simulink model "IBR_Control_Benchmark_2024b"  (R2024b)
settings: Solver=ode4  StartTime=0.0  StopTime=1  FixedStep=5e-5  RelTol=1e-3
values from neighbouring files (symbols this model uses):
  Ki_I = Simulink.Parameter    [IBR_Control_Parameters.m]
  Ki_PLL = Simulink.Parameter    [IBR_Control_Parameters.m]
  Kp_I = Simulink.Parameter    [IBR_Control_Parameters.m]
  Kp_PLL = Simulink.Parameter    [IBR_Control_Parameters.m]
  Lc = Simulink.Parameter    [IBR_Control_Parameters.m]
  Pref = Simulink.Parameter    [IBR_Control_Parameters.m]
  Qref = Simulink.Parameter    [IBR_Control_Parameters.m]
  Rc = Simulink.Parameter    [IBR_Control_Parameters.m]
  Re = Vn^2 / Sk / sqrt(RXratio^2 + 1) * RXratio    [IBR_Control_Parameters.m]
  Vn = 400e3    (= 400000)    [IBR_Control_Parameters.m]
undefined symbols (not defined in the file or in its folder): cVc, DiscIntNeverNeededParam, dspblkCoreblockFVToolHelper, fn, gcbh, ia0, ib0, ic0, id0, iq0, Kp_S, Le, T_S, theta0
libraries: slpidlib x3, model_info x1
settings Model: ParamWorkspaceSource=ReferencedWorkspace  Creator=evansolingen  LastModifiedBy=if47izeq
settings DataIOCC: LimitDataPoints=on  SaveFormat=Array  SignalLoggingSaveFormat=ModelDataLogs  SaveOutput=off  SignalLogging=off  SaveTime=off  ReturnWorkspaceOutputs=off
settings OptimizationCC: EnhancedBackFolding=on  ExpressionFolding=off  PassReuseOutputArgsThreshold=0  ExpressionDepthLimit=2147483647  OptimizeBlockOrder=speed  DifferentSizesBufferReuse=on
settings DebuggingCC: UnderspecifiedInitializationDetection=Classic  MergeDetectMultiDrivingBlocksExec=none  SolverPrmCheckMsg=warning  MultiTaskDSMMsg=warning  MultiTaskCondExecSysMsg=none  ParameterTunabilityLossMsg=error  FcnCallInpInsideContextMsg=warning  UnconnectedInputMsg=warning  UnconnectedOutputMsg=warning  UnconnectedLineMsg=warning  AllowSymbolicDim=off  StateNameClashWarn=warning  SFUnexpectedBacktrackingDiag=warning  SFNoUnconditionalDefaultTransitionDiag=warning  SFExecutionAtInitializationDiag=none  UnderSpecifiedDimensionMsg=warning  ArithmeticOperatorsInVariantConditions=warning
settings HardwareCC: ProdBitPerPointer=32  ProdBitPerSizeT=32  ProdBitPerPtrDiffT=32  ProdLargestAtomicFloat=None  ProdIntDivRoundTo=Undefined  ProdEndianess=Unspecified  ProdWordSize=32  ProdHWDeviceType=32-bit Generic
settings ModelReferenceCC: UpdateModelReferenceTargets=Force  EnableRefExpFcnMdlSchedulingChecks=on  PropagateSignalLabelsOutOfModel=off
settings SFSimCC: SimUseLocalCustomCode=off  SimParseCustomCode=off  MATLABDynamicMemAlloc=off  CustomCodeUndefinedFunction=UseInterfaceOnly
settings RTWCC: Description=Create Visual C/C++ Solution File for Simulink Coder  SystemTargetFile=IEC61400_27_DLL.tlc  TemplateMakefile=IEC61400_27_DLL.tmf  RTWUseLocalCustomCode=off  GPUComputeCapability=3.5
settings CodeAppCC: ForceParamTrailComments=on  OperatorAnnotations=on
settings STFCustomTargetCC: ModelReferenceCompliant=off  MATLABClassNameForMDSCustomization=Simulink.SoftwareTarget.TargetSpecificTriggerConfigurationBase  GRTInterface=on  SystemTargetFile=IEC61400_27_DLL.tlc
settings ConfigComp: CovMetricSettings=dw  CovSaveCumulativeToWorkspaceVar=on  CovSaveSingleToWorkspaceVar=on  CovExternalEMLEnable=off

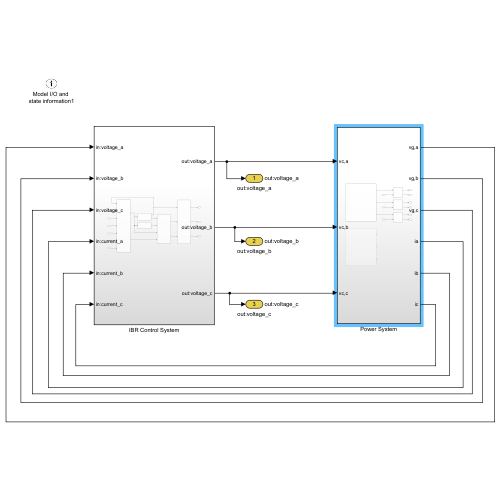
[thumbnail: Simulink's stored preview of the top-level diagram]
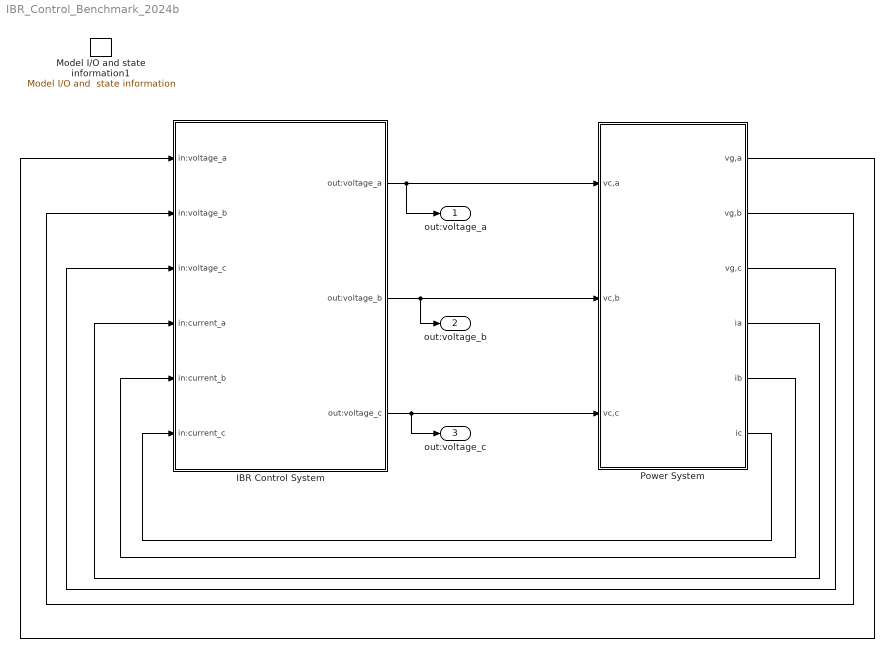
== system IBR_Control_Benchmark_2024b ==
  IBR Control System : Subsystem
  Model I/O and state information1 : model_info/Model I//O and  state information
  Power System : Subsystem
  out:voltage_a : Outport  SignalName=out:voltage_a
  out:voltage_b : Outport  Port=2  SignalName=out:voltage_b
  out:voltage_c : Outport  Port=3  SignalName=out:voltage_c
  wires:
  IBR Control System/1(out:voltage_a) -> out:voltage_a/1, Power System/1(vc,a)
  IBR Control System/2(out:voltage_b) -> out:voltage_b/1, Power System/2(vc,b)
  IBR Control System/3(out:voltage_c) -> out:voltage_c/1, Power System/3(vc,c)
  Power System/6(ic) -> IBR Control System/6(in:current_c)
  Power System/5(ib) -> IBR Control System/5(in:current_b)
  Power System/4(ia) -> IBR Control System/4(in:current_a)
  Power System/3(vg,c) -> IBR Control System/3(in:voltage_c)
  Power System/2(vg,b) -> IBR Control System/2(in:voltage_b)
  Power System/1(vg,a) -> IBR Control System/1(in:voltage_a)

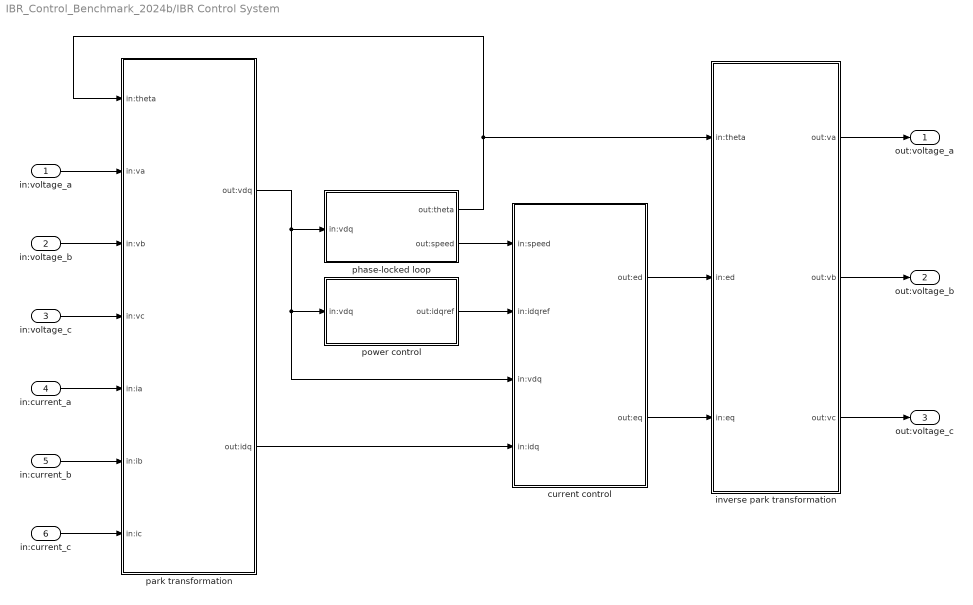
== system IBR_Control_Benchmark_2024b/IBR Control System ==
  in:voltage_a : Inport
  in:voltage_b : Inport  Port=2
  in:voltage_c : Inport  Port=3
  in:current_a : Inport  Port=4
  in:current_b : Inport  Port=5
  in:current_c : Inport  Port=6
  current control : Subsystem
  inverse park transformation : Subsystem
  park transformation : Subsystem
  phase-locked loop : Subsystem
  power control : Subsystem
  out:voltage_a : Outport
  out:voltage_b : Outport  Port=2
  out:voltage_c : Outport  Port=3
  wires:
  in:current_b/1 -> park transformation/6(in:ib)
  in:current_c/1 -> park transformation/7(in:ic)
  in:current_a/1 -> park transformation/5(in:ia)
  in:voltage_a/1 -> park transformation/2(in:va)
  in:voltage_b/1 -> park transformation/3(in:vb)
  in:voltage_c/1 -> park transformation/4(in:vc)
  park transformation/1(out:vdq) -> current control/3(in:vdq), power control/1(in:vdq), phase-locked loop/1(in:vdq)
  park transformation/2(out:idq) -> current control/4(in:idq)
  phase-locked loop/2(out:speed) -> current control/1(in:speed)
  power control/1(out:idqref) -> current control/2(in:idqref)
  current control/1(out:ed) -> inverse park transformation/2(in:ed)
  current control/2(out:eq) -> inverse park transformation/3(in:eq)
  inverse park transformation/1(out:va) -> out:voltage_a/1
  inverse park transformation/2(out:vb) -> out:voltage_b/1
  inverse park transformation/3(out:vc) -> out:voltage_c/1
  phase-locked loop/1(out:theta) -> park transformation/1(in:theta), inverse park transformation/1(in:theta)

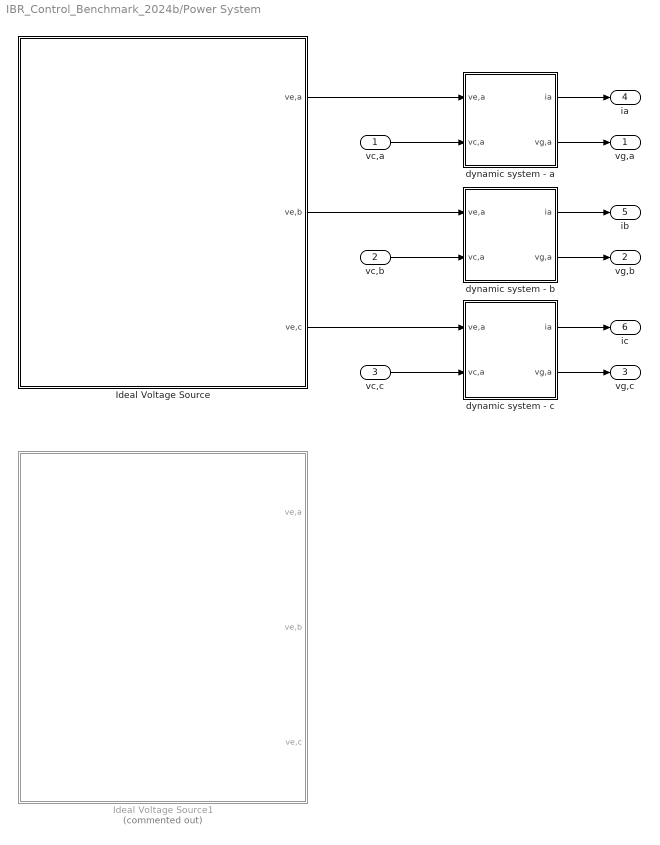
== system IBR_Control_Benchmark_2024b/Power System ==
  vc,a : Inport
  vc,b : Inport  Port=2
  vc,c : Inport  Port=3
  Ideal Voltage Source : Subsystem
  Ideal Voltage Source1 : Subsystem  Commented=on
  dynamic system - a : Subsystem
  dynamic system - b : Subsystem
  dynamic system - c : Subsystem
  vg,a : Outport
  vg,b : Outport  Port=2
  vg,c : Outport  Port=3
  ia : Outport  Port=4
  ib : Outport  Port=5
  ic : Outport  Port=6
  wires:
  Ideal Voltage Source/2(ve,b) -> dynamic system - b/1(ve,a)
  Ideal Voltage Source/1(ve,a) -> dynamic system - a/1(ve,a)
  Ideal Voltage Source/3(ve,c) -> dynamic system - c/1(ve,a)
  dynamic system - a/2(vg,a) -> vg,a/1
  dynamic system - a/1(ia) -> ia/1
  dynamic system - b/1(ia) -> ib/1
  dynamic system - c/1(ia) -> ic/1
  dynamic system - c/2(vg,a) -> vg,c/1
  dynamic system - b/2(vg,a) -> vg,b/1
  vc,a/1 -> dynamic system - a/2(vc,a)
  vc,b/1 -> dynamic system - b/2(vc,a)
  vc,c/1 -> dynamic system - c/2(vc,a)

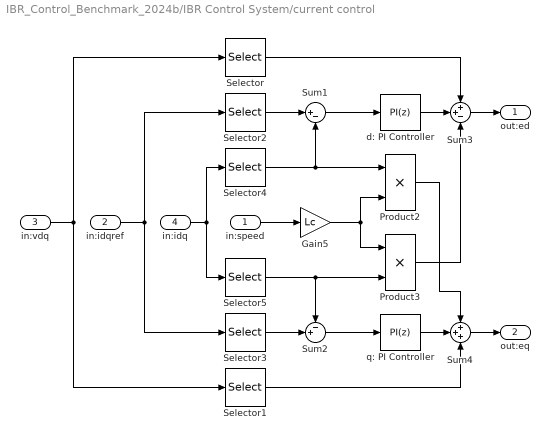
== system IBR_Control_Benchmark_2024b/IBR Control System/current control ==
  in:speed : Inport
  in:idqref : Inport  Port=2
  in:vdq : Inport  Port=3
  in:idq : Inport  Port=4
  Gain5 : Gain  Gain=Lc
  Product2 : Product
  Product3 : Product
  Selector : Selector  InputPortWidth=2  IndexOptions=Index vector (dialog)  Indices=1  OutputSizes=1
  Selector1 : Selector  InputPortWidth=2  IndexOptions=Index vector (dialog)  Indices=[2]  OutputSizes=1
  Selector2 : Selector  InputPortWidth=2  IndexOptions=Index vector (dialog)  Indices=[1]  OutputSizes=1
  Selector3 : Selector  InputPortWidth=2  IndexOptions=Index vector (dialog)  Indices=[2]  OutputSizes=1
  Selector4 : Selector  InputPortWidth=2  IndexOptions=Index vector (dialog)  Indices=[1]  OutputSizes=1
  Selector5 : Selector  InputPortWidth=2  IndexOptions=Index vector (dialog)  Indices=[2]  OutputSizes=1
  Sum1 : Sum  Inputs=|+-
  Sum2 : Sum  Inputs=-+|
  Sum3 : Sum  Inputs=++-
  Sum4 : Sum  Inputs=+++
  d: PI Controller : slpidlib/PID Controller  Controller=PI  Form=Parallel  TimeDomain=Discrete-time  UseExternalTs=off  SampleTime=-1  IntegratorMethod=Forward Euler  FilterMethod=Forward Euler  ControllerParametersSource=internal  P=Kp_I  I=Ki_I  UseKiTs=off  D=0  UseExternalDerivativeSource=off  N=100  UseFilter=on  TunerSelectOption=Transfer Function Based (PID Tuner App)  InitialConditionSource=internal  InitialConditionForIntegrator=xid0  InitialConditionForFilter=0  DifferentiatorICPrevScaledInput=0  ExternalReset=none  TrackingMode=off  Kt=1  LimitOutput=off  SatLimitsSource=internal  UpperSaturationLimit=inf  LowerSaturationLimit=-inf  LinearizeAsGain=on  AntiWindupMode=none  Kb=1  LimitIntegrator=off  UpperIntegratorSaturationLimit=inf  LowerIntegratorSaturationLimit=-inf  POutMin=[]  POutMax=[]  IOutMin=[]  IOutMax=[]  DOutMin=[]  DOutMax=[]  NOutMin=[]  NOutMax=[]  SumOutMin=[]  SumOutMax=[]  SaturationOutMin=[]  SaturationOutMax=[]  PParamMin=[]  PParamMax=[]  IParamMin=[]  IParamMax=[]  DParamMin=[]  DParamMax=[]  NParamMin=[]  NParamMax=[]  KbParamMin=[]  KbParamMax=[]  KtParamMin=[]  KtParamMax=[]  KbOutMin=[]  KbOutMax=[]  KtOutMin=[]  KtOutMax=[]  IntegratorOutMin=[]  IntegratorOutMax=[]  FilterOutMin=[]  FilterOutMax=[]  SumI1OutMin=[]  SumI1OutMax=[]  SumI2OutMin=[]  SumI2OutMax=[]  SumI3OutMin=[]  SumI3OutMax=[]  SumI4OutMin=[]  SumI4OutMax=[]  SumDOutMin=[]  SumDOutMax=[]  DifferentiatorOutMin=[]  DifferentiatorOutMax=[]  FilterDiffOutCoefMin=[]  FilterDiffOutCoefMax=[]  ReciprocalOutMin=[]  ReciprocalOutMax=[]  SumDenOutMin=[]  SumDenOutMax=[]  SumNumOutMin=[]  SumNumOutMax=[]  DivideOutMin=[]  DivideOutMax=[]  UdiffTsProdOutMin=[]  UdiffTsProdOutMax=[]  NTsProdOutMin=[]  NTsProdOutMax=[]  UintegralTsProdOutMin=[]  UintegralTsProdOutMax=[]  UngainTsProdOutMin=[]  UngainTsProdOutMax=[]  ClampingZeroOutDataTypeStr=Inherit: Inherit via back propagation  ClampingZeroOutMin=[]  ClampingZeroOutMax=[]  FilterDenConstantOutDataTypeStr=Inherit: Inherit via back propagation  FilterDenConstantOutMin=[]  FilterDenConstantOutMax=[]  PCopyOutDataTypeStr=Inherit: Inherit via back propagation  PCopyOutMin=[]  PCopyOutMax=[]  NCopyOutDataTypeStr=Inherit: Inherit via back propagation  NCopyOutMin=[]  NCopyOutMax=[]  IntegratorContinuousStateAttributes=''  IntegratorStateMustResolveToSignalObject=off  IntegratorRTWStateStorageClass=Auto  FilterContinuousStateAttributes=''  FilterStateMustResolveToSignalObject=off  FilterRTWStateStorageClass=Auto  ParallelPVariant=InternalParameters  IdealPVariant=Disabled  IVariant=InternalParameters  DVariant=Disabled  IntegratorVariant=Discrete  SatVariant=Disabled  AWVariant=Passthrough  PCopyVariant=Disabled  TRVariant=Disabled  FdbkBlocksVariant=Forward  IdealPFdbkVariant=Disabled  SatFdbkVariant=Disabled  DerivativeFilterVariant=Disabled  NVariant=Disabled  NCopyVariant=Disabled_SignalSpec  FilterICVariant=Disabled  IntegratorICVariant=InternalICs  ExternalResetVariant=Disabled  TRSumVariant=Passthrough  SumFdbkVariant=Disabled  SumVariant=Sum_PI  TsampFilterVariant=InternalTs  TsampNgainVariant=Passthrough  TsampIntegralVariant=Disabled_SignalSpec  ExternalSaturationOutDataTypeStr=Inherit: Same as second input  DerivativeSourceVariant=Disabled  PreIntVariant=InternalPreInt
  q: PI Controller : slpidlib/PID Controller  Controller=PI  Form=Parallel  TimeDomain=Discrete-time  UseExternalTs=off  SampleTime=-1  IntegratorMethod=Forward Euler  FilterMethod=Forward Euler  ControllerParametersSource=internal  P=Kp_I  I=Ki_I  UseKiTs=off  D=0  UseExternalDerivativeSource=off  N=100  UseFilter=on  TunerSelectOption=Transfer Function Based (PID Tuner App)  InitialConditionSource=internal  InitialConditionForIntegrator=xiq0  InitialConditionForFilter=0  DifferentiatorICPrevScaledInput=0  ExternalReset=none  TrackingMode=off  Kt=1  LimitOutput=off  SatLimitsSource=internal  UpperSaturationLimit=inf  LowerSaturationLimit=-inf  LinearizeAsGain=on  AntiWindupMode=none  Kb=1  LimitIntegrator=off  UpperIntegratorSaturationLimit=inf  LowerIntegratorSaturationLimit=-inf  POutMin=[]  POutMax=[]  IOutMin=[]  IOutMax=[]  DOutMin=[]  DOutMax=[]  NOutMin=[]  NOutMax=[]  SumOutMin=[]  SumOutMax=[]  SaturationOutMin=[]  SaturationOutMax=[]  PParamMin=[]  PParamMax=[]  IParamMin=[]  IParamMax=[]  DParamMin=[]  DParamMax=[]  NParamMin=[]  NParamMax=[]  KbParamMin=[]  KbParamMax=[]  KtParamMin=[]  KtParamMax=[]  KbOutMin=[]  KbOutMax=[]  KtOutMin=[]  KtOutMax=[]  IntegratorOutMin=[]  IntegratorOutMax=[]  FilterOutMin=[]  FilterOutMax=[]  SumI1OutMin=[]  SumI1OutMax=[]  SumI2OutMin=[]  SumI2OutMax=[]  SumI3OutMin=[]  SumI3OutMax=[]  SumI4OutMin=[]  SumI4OutMax=[]  SumDOutMin=[]  SumDOutMax=[]  DifferentiatorOutMin=[]  DifferentiatorOutMax=[]  FilterDiffOutCoefMin=[]  FilterDiffOutCoefMax=[]  ReciprocalOutMin=[]  ReciprocalOutMax=[]  SumDenOutMin=[]  SumDenOutMax=[]  SumNumOutMin=[]  SumNumOutMax=[]  DivideOutMin=[]  DivideOutMax=[]  UdiffTsProdOutMin=[]  UdiffTsProdOutMax=[]  NTsProdOutMin=[]  NTsProdOutMax=[]  UintegralTsProdOutMin=[]  UintegralTsProdOutMax=[]  UngainTsProdOutMin=[]  UngainTsProdOutMax=[]  ClampingZeroOutDataTypeStr=Inherit: Inherit via back propagation  ClampingZeroOutMin=[]  ClampingZeroOutMax=[]  FilterDenConstantOutDataTypeStr=Inherit: Inherit via back propagation  FilterDenConstantOutMin=[]  FilterDenConstantOutMax=[]  PCopyOutDataTypeStr=Inherit: Inherit via back propagation  PCopyOutMin=[]  PCopyOutMax=[]  NCopyOutDataTypeStr=Inherit: Inherit via back propagation  NCopyOutMin=[]  NCopyOutMax=[]  IntegratorContinuousStateAttributes=''  IntegratorStateMustResolveToSignalObject=off  IntegratorRTWStateStorageClass=Auto  FilterContinuousStateAttributes=''  FilterStateMustResolveToSignalObject=off  FilterRTWStateStorageClass=Auto  ParallelPVariant=InternalParameters  IdealPVariant=Disabled  IVariant=InternalParameters  DVariant=Disabled  IntegratorVariant=Discrete  SatVariant=Disabled  AWVariant=Passthrough  PCopyVariant=Disabled  TRVariant=Disabled  FdbkBlocksVariant=Forward  IdealPFdbkVariant=Disabled  SatFdbkVariant=Disabled  DerivativeFilterVariant=Disabled  NVariant=Disabled  NCopyVariant=Disabled_SignalSpec  FilterICVariant=Disabled  IntegratorICVariant=InternalICs  ExternalResetVariant=Disabled  TRSumVariant=Passthrough  SumFdbkVariant=Disabled  SumVariant=Sum_PI  TsampFilterVariant=InternalTs  TsampNgainVariant=Passthrough  TsampIntegralVariant=Disabled_SignalSpec  ExternalSaturationOutDataTypeStr=Inherit: Same as second input  DerivativeSourceVariant=Disabled  PreIntVariant=InternalPreInt
  out:ed : Outport
  out:eq : Outport  Port=2
  wires:
  Gain5/1 -> Product2/2, Product3/1
  Sum4/1 -> out:eq/1
  Product3/1 -> Sum3/3
  Selector3/1 -> Sum2/2
  Sum1/1 -> d: PI Controller/1
  Sum3/1 -> out:ed/1
  Product2/1 -> Sum4/1
  Sum2/1 -> q: PI Controller/1
  in:speed/1 -> Gain5/1
  in:vdq/1 -> Selector1/1, Selector/1
  in:idq/1 -> Selector5/1, Selector4/1
  Selector5/1 -> Product3/2, Sum2/1
  d: PI Controller/1 -> Sum3/2
  q: PI Controller/1 -> Sum4/2
  Selector1/1 -> Sum4/3
  in:idqref/1 -> Selector2/1, Selector3/1
  Selector2/1 -> Sum1/1
  Selector/1 -> Sum3/1
  Selector4/1 -> Product2/1, Sum1/2

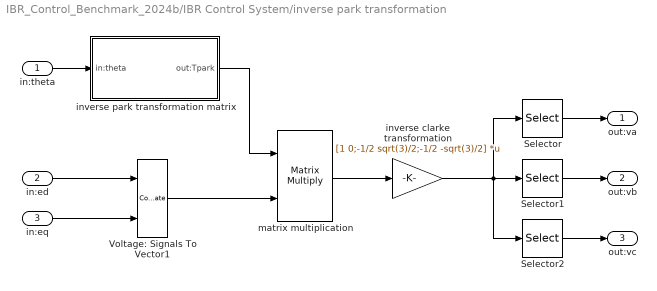
== system IBR_Control_Benchmark_2024b/IBR Control System/inverse park transformation ==
  in:theta : Inport
  in:ed : Inport  Port=2
  in:eq : Inport  Port=3
  Selector : Selector  InputPortWidth=3  IndexOptions=Index vector (dialog)  Indices=[1]  OutputSizes=1
  Selector1 : Selector  InputPortWidth=3  IndexOptions=Index vector (dialog)  Indices=[2]  OutputSizes=1
  Selector2 : Selector  InputPortWidth=3  IndexOptions=Index vector (dialog)  Indices=[3]  OutputSizes=1
  Voltage: Signals To Vector1 : Concatenate  Mode=Multidimensional array
  inverse clarke transformation : Gain  Gain=[1 0;-1/2 sqrt(3)/2;-1/2 -sqrt(3)/2]  Multiplication=Matrix(K*u)
  inverse park transformation matrix : Subsystem
  matrix multiplication : Product  Multiplication=Matrix(*)
  out:va : Outport
  out:vb : Outport  Port=2
  out:vc : Outport  Port=3
  wires:
  inverse park transformation matrix/1(out:Tpark) -> matrix multiplication/1
  in:theta/1 -> inverse park transformation matrix/1(in:theta)
  inverse clarke transformation/1 -> Selector2/1, Selector1/1, Selector/1
  matrix multiplication/1 -> inverse clarke transformation/1
  Selector1/1 -> out:vb/1
  Selector/1 -> out:va/1
  in:ed/1 -> Voltage: Signals To Vector1/1
  in:eq/1 -> Voltage: Signals To Vector1/2
  Voltage: Signals To Vector1/1 -> matrix multiplication/2
  Selector2/1 -> out:vc/1

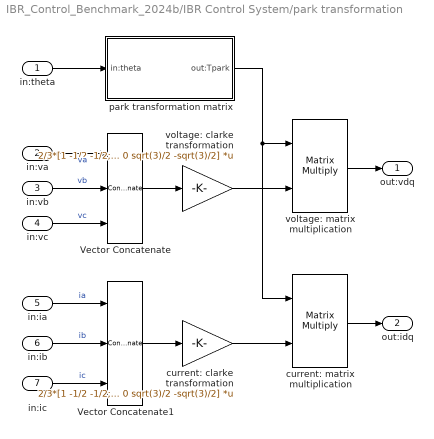
== system IBR_Control_Benchmark_2024b/IBR Control System/park transformation ==
  in:theta : Inport
  in:va : Inport  Port=2
  in:vb : Inport  Port=3
  in:vc : Inport  Port=4
  in:ia : Inport  Port=5
  in:ib : Inport  Port=6
  in:ic : Inport  Port=7
  Vector Concatenate : Concatenate  NumInputs=3  Mode=Multidimensional array
  Vector Concatenate1 : Concatenate  NumInputs=3  Mode=Multidimensional array
  current: clarke transformation : Gain  Gain=2/3*[1 -1/2 -1/2; 0 sqrt(3)/2 -sqrt(3)/2]  Multiplication=Matrix(K*u)
  current: matrix multiplication : Product  Multiplication=Matrix(*)
  park transformation matrix : Subsystem
  voltage: clarke transformation : Gain  Gain=2/3*[1 -1/2 -1/2; 0 sqrt(3)/2 -sqrt(3)/2]  Multiplication=Matrix(K*u)
  voltage: matrix multiplication : Product  Multiplication=Matrix(*)
  out:vdq : Outport
  out:idq : Outport  Port=2
  wires:
  in:va/1 -> Vector Concatenate/1  "va"
  in:ib/1 -> Vector Concatenate1/2  "ib"
  in:ic/1 -> Vector Concatenate1/3  "ic"
  Vector Concatenate1/1 -> current: clarke transformation/1
  in:ia/1 -> Vector Concatenate1/1  "ia"
  voltage: matrix multiplication/1 -> out:vdq/1
  in:vb/1 -> Vector Concatenate/2  "vb"
  in:vc/1 -> Vector Concatenate/3  "vc"
  Vector Concatenate/1 -> voltage: clarke transformation/1
  voltage: clarke transformation/1 -> voltage: matrix multiplication/2
  current: clarke transformation/1 -> current: matrix multiplication/2
  in:theta/1 -> park transformation matrix/1(in:theta)
  park transformation matrix/1(out:Tpark) -> voltage: matrix multiplication/1, current: matrix multiplication/1
  current: matrix multiplication/1 -> out:idq/1

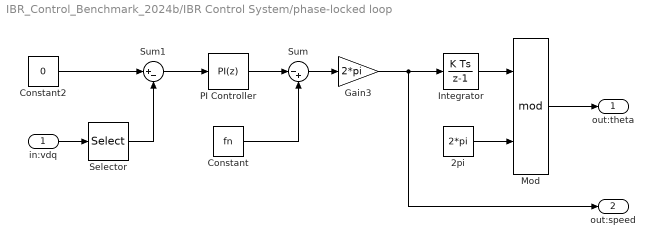
== system IBR_Control_Benchmark_2024b/IBR Control System/phase-locked loop ==
  in:vdq : Inport
  2pi : Constant  Value=2*pi
  Constant : Constant  Value=fn
  Constant2 : Constant  Value=0
  Gain3 : Gain  Gain=2*pi
  Integrator : DiscreteIntegrator  InitialCondition=theta0  SampleTime=-1  ICPrevOutput=DiscIntNeverNeededParam  ICPrevScaledInput=DiscIntNeverNeededParam
  Mod : Math  Operator=mod
  PI Controller : slpidlib/PID Controller  Controller=PI  Form=Parallel  TimeDomain=Discrete-time  UseExternalTs=off  SampleTime=-1  IntegratorMethod=Forward Euler  FilterMethod=Forward Euler  ControllerParametersSource=internal  P=Kp_PLL  I=Ki_PLL  UseKiTs=off  D=0  UseExternalDerivativeSource=off  N=100  UseFilter=on  TunerSelectOption=Transfer Function Based (PID Tuner App)  InitialConditionSource=internal  InitialConditionForIntegrator=0  InitialConditionForFilter=0  DifferentiatorICPrevScaledInput=0  ExternalReset=none  TrackingMode=off  Kt=1  LimitOutput=off  SatLimitsSource=internal  UpperSaturationLimit=inf  LowerSaturationLimit=-inf  LinearizeAsGain=on  AntiWindupMode=none  Kb=1  LimitIntegrator=off  UpperIntegratorSaturationLimit=inf  LowerIntegratorSaturationLimit=-inf  POutMin=[]  POutMax=[]  IOutMin=[]  IOutMax=[]  DOutMin=[]  DOutMax=[]  NOutMin=[]  NOutMax=[]  SumOutMin=[]  SumOutMax=[]  SaturationOutMin=[]  SaturationOutMax=[]  PParamMin=[]  PParamMax=[]  IParamMin=[]  IParamMax=[]  DParamMin=[]  DParamMax=[]  NParamMin=[]  NParamMax=[]  KbParamMin=[]  KbParamMax=[]  KtParamMin=[]  KtParamMax=[]  KbOutMin=[]  KbOutMax=[]  KtOutMin=[]  KtOutMax=[]  IntegratorOutMin=[]  IntegratorOutMax=[]  FilterOutMin=[]  FilterOutMax=[]  SumI1OutMin=[]  SumI1OutMax=[]  SumI2OutMin=[]  SumI2OutMax=[]  SumI3OutMin=[]  SumI3OutMax=[]  SumI4OutMin=[]  SumI4OutMax=[]  SumDOutMin=[]  SumDOutMax=[]  DifferentiatorOutMin=[]  DifferentiatorOutMax=[]  FilterDiffOutCoefMin=[]  FilterDiffOutCoefMax=[]  ReciprocalOutMin=[]  ReciprocalOutMax=[]  SumDenOutMin=[]  SumDenOutMax=[]  SumNumOutMin=[]  SumNumOutMax=[]  DivideOutMin=[]  DivideOutMax=[]  UdiffTsProdOutMin=[]  UdiffTsProdOutMax=[]  NTsProdOutMin=[]  NTsProdOutMax=[]  UintegralTsProdOutMin=[]  UintegralTsProdOutMax=[]  UngainTsProdOutMin=[]  UngainTsProdOutMax=[]  ClampingZeroOutDataTypeStr=Inherit: Inherit via back propagation  ClampingZeroOutMin=[]  ClampingZeroOutMax=[]  FilterDenConstantOutDataTypeStr=Inherit: Inherit via back propagation  FilterDenConstantOutMin=[]  FilterDenConstantOutMax=[]  PCopyOutDataTypeStr=Inherit: Inherit via back propagation  PCopyOutMin=[]  PCopyOutMax=[]  NCopyOutDataTypeStr=Inherit: Inherit via back propagation  NCopyOutMin=[]  NCopyOutMax=[]  IntegratorContinuousStateAttributes=''  IntegratorStateMustResolveToSignalObject=off  IntegratorRTWStateStorageClass=Auto  FilterContinuousStateAttributes=''  FilterStateMustResolveToSignalObject=off  FilterRTWStateStorageClass=Auto  ParallelPVariant=InternalParameters  IdealPVariant=Disabled  IVariant=InternalParameters  DVariant=Disabled  IntegratorVariant=Discrete  SatVariant=Disabled  AWVariant=Passthrough  PCopyVariant=Disabled  TRVariant=Disabled  FdbkBlocksVariant=Forward  IdealPFdbkVariant=Disabled  SatFdbkVariant=Disabled  DerivativeFilterVariant=Disabled  NVariant=Disabled  NCopyVariant=Disabled_SignalSpec  FilterICVariant=Disabled  IntegratorICVariant=InternalICs  ExternalResetVariant=Disabled  TRSumVariant=Passthrough  SumFdbkVariant=Disabled  SumVariant=Sum_PI  TsampFilterVariant=InternalTs  TsampNgainVariant=Passthrough  TsampIntegralVariant=Disabled_SignalSpec  ExternalSaturationOutDataTypeStr=Inherit: Same as second input  DerivativeSourceVariant=Disabled  PreIntVariant=InternalPreInt
  Selector : Selector  InputPortWidth=2  IndexOptions=Index vector (dialog)  Indices=[2]  OutputSizes=1
  Sum : Sum  Inputs=|-+
  Sum1 : Sum  Inputs=|+-
  out:theta : Outport
  out:speed : Outport  Port=2
  wires:
  Constant/1 -> Sum/2
  Sum/1 -> Gain3/1
  2pi/1 -> Mod/2
  Gain3/1 -> out:speed/1, Integrator/1
  Sum1/1 -> PI Controller/1
  Mod/1 -> out:theta/1
  in:vdq/1 -> Selector/1
  Selector/1 -> Sum1/2
  Constant2/1 -> Sum1/1
  PI Controller/1 -> Sum/1
  Integrator/1 -> Mod/1

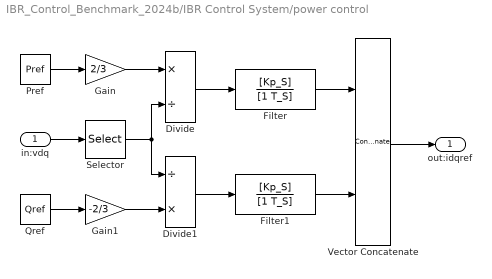
== system IBR_Control_Benchmark_2024b/IBR Control System/power control ==
  in:vdq : Inport
  Divide : Product  Inputs=*/
  Divide1 : Product  Inputs=/*
  Filter : DiscreteTransferFcn  LoadFcn=dspblkCoreblockFVToolHelper(gcbh,'load');  Numerator=[Kp_S]  Denominator=[1 T_S]  InitialStates=id0/Kp_S
      settings: CopyFcn=dspblkCoreblockFVToolHelper(gcbh,'copy');  DeleteFcn=dspblkCoreblockFVToolHelper(gcbh,'close');  ModelCloseFcn=dspblkCoreblockFVToolHelper(gcbh,'close');  PreSaveFcn=dspblkCoreblockFVToolHelper(gcbh,'presave');  PostSaveFcn=dspblkCoreblockFVToolHelper(gcbh,'postsave');  CloseFcn=dspblkCoreblockFVToolHelper(gcbh,'close');
  Filter1 : DiscreteTransferFcn  LoadFcn=dspblkCoreblockFVToolHelper(gcbh,'load');  Numerator=[Kp_S]  Denominator=[1 T_S]  InitialStates=iq0/Kp_S
      settings: CopyFcn=dspblkCoreblockFVToolHelper(gcbh,'copy');  DeleteFcn=dspblkCoreblockFVToolHelper(gcbh,'close');  ModelCloseFcn=dspblkCoreblockFVToolHelper(gcbh,'close');  PreSaveFcn=dspblkCoreblockFVToolHelper(gcbh,'presave');  PostSaveFcn=dspblkCoreblockFVToolHelper(gcbh,'postsave');  CloseFcn=dspblkCoreblockFVToolHelper(gcbh,'close');
  Gain : Gain  Gain=2/3
  Gain1 : Gain  Gain=-2/3
  Pref : Constant  Value=Pref
  Qref : Constant  Value=Qref
  Selector : Selector  InputPortWidth=2  IndexOptions=Index vector (dialog)  Indices=[1]  OutputSizes=1
  Vector Concatenate : Concatenate  Mode=Multidimensional array
  out:idqref : Outport
  wires:
  Pref/1 -> Gain/1
  Gain/1 -> Divide/1
  Qref/1 -> Gain1/1
  Selector/1 -> Divide/2, Divide1/1
  Gain1/1 -> Divide1/2
  Divide1/1 -> Filter1/1
  Divide/1 -> Filter/1
  Filter/1 -> Vector Concatenate/1
  Filter1/1 -> Vector Concatenate/2
  in:vdq/1 -> Selector/1
  Vector Concatenate/1 -> out:idqref/1

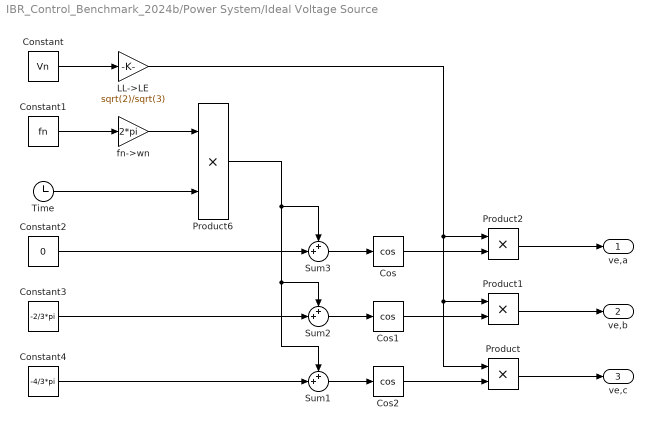
== system IBR_Control_Benchmark_2024b/Power System/Ideal Voltage Source ==
  Constant : Constant  Value=Vn
  Constant1 : Constant  Value=fn
  Constant2 : Constant  Value=0
  Constant3 : Constant  Value=-2/3*pi
  Constant4 : Constant  Value=-4/3*pi
  Cos : Trigonometry  Operator=cos
  Cos1 : Trigonometry  Operator=cos
  Cos2 : Trigonometry  Operator=cos
  LL->LE : Gain  Gain=sqrt(2)/sqrt(3)
  Product{,1..2,6} (4 alike) : Product
  Sum1 : Sum  Inputs=++|
  Sum2 : Sum  Inputs=++|
  Sum3 : Sum  Inputs=++|
  Time : Clock
  fn->wn : Gain  Gain=2*pi
  ve,a : Outport
  ve,b : Outport  Port=2
  ve,c : Outport  Port=3
  wires:
  Product/1 -> ve,c/1
  Cos1/1 -> Product1/2
  Product6/1 -> Sum1/1, Sum2/1, Sum3/1
  Cos/1 -> Product2/2
  Sum3/1 -> Cos/1
  LL->LE/1 -> Product1/1, Product/1, Product2/1
  Constant3/1 -> Sum2/2
  Constant/1 -> LL->LE/1
  Cos2/1 -> Product/2
  Sum1/1 -> Cos2/1
  Time/1 -> Product6/2
  Sum2/1 -> Cos1/1
  Constant2/1 -> Sum3/2
  fn->wn/1 -> Product6/1
  Constant4/1 -> Sum1/2
  Constant1/1 -> fn->wn/1
  Product1/1 -> ve,b/1
  Product2/1 -> ve,a/1

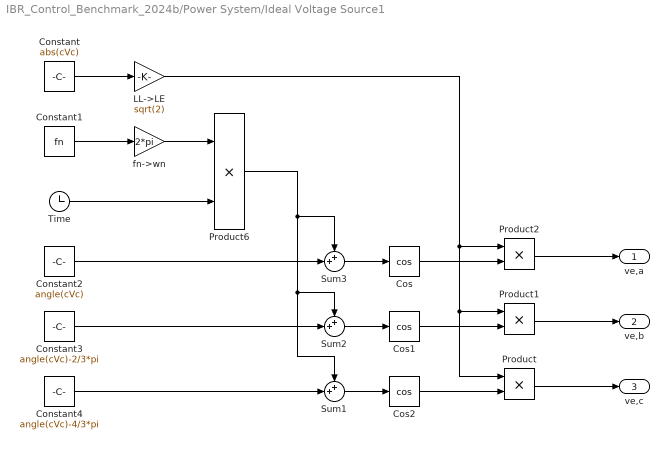
== system IBR_Control_Benchmark_2024b/Power System/Ideal Voltage Source1 ==
  Constant : Constant  Value=abs(cVc)
  Constant1 : Constant  Value=fn
  Constant2 : Constant  Value=angle(cVc)
  Constant3 : Constant  Value=angle(cVc)-2/3*pi
  Constant4 : Constant  Value=angle(cVc)-4/3*pi
  Cos : Trigonometry  Operator=cos
  Cos1 : Trigonometry  Operator=cos
  Cos2 : Trigonometry  Operator=cos
  LL->LE : Gain  Gain=sqrt(2)
  Product{,1..2,6} (4 alike) : Product
  Sum1 : Sum  Inputs=++|
  Sum2 : Sum  Inputs=++|
  Sum3 : Sum  Inputs=++|
  Time : Clock
  fn->wn : Gain  Gain=2*pi
  ve,a : Outport
  ve,b : Outport  Port=2
  ve,c : Outport  Port=3
  wires:
  Product/1 -> ve,c/1
  Cos1/1 -> Product1/2
  Product6/1 -> Sum1/1, Sum2/1, Sum3/1
  Cos/1 -> Product2/2
  Sum3/1 -> Cos/1
  LL->LE/1 -> Product1/1, Product/1, Product2/1
  Constant3/1 -> Sum2/2
  Constant/1 -> LL->LE/1
  Cos2/1 -> Product/2
  Sum1/1 -> Cos2/1
  Time/1 -> Product6/2
  Sum2/1 -> Cos1/1
  Constant2/1 -> Sum3/2
  fn->wn/1 -> Product6/1
  Constant4/1 -> Sum1/2
  Constant1/1 -> fn->wn/1
  Product1/1 -> ve,b/1
  Product2/1 -> ve,a/1

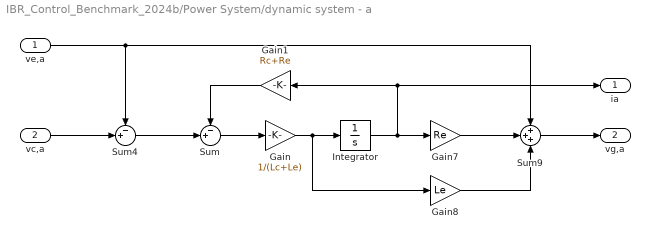
== system IBR_Control_Benchmark_2024b/Power System/dynamic system - a ==
  ve,a : Inport
  vc,a : Inport  Port=2
  Gain : Gain  Gain=1/(Lc+Le)
  Gain1 : Gain  Gain=Rc+Re
  Gain7 : Gain  Gain=Re
  Gain8 : Gain  Gain=Le
  Integrator : Integrator  InitialCondition=ia0
  Sum : Sum  Inputs=-+|
  Sum4 : Sum  Inputs=-+|
  Sum9 : Sum  Inputs=+++
  ia : Outport
  vg,a : Outport  Port=2
  wires:
  Gain/1 -> Integrator/1, Gain8/1
  Gain7/1 -> Sum9/2
  vc,a/1 -> Sum4/2
  Gain8/1 -> Sum9/3
  Integrator/1 -> ia/1, Gain1/1, Gain7/1
  ve,a/1 -> Sum9/1, Sum4/1
  Sum9/1 -> vg,a/1
  Sum/1 -> Gain/1
  Gain1/1 -> Sum/1
  Sum4/1 -> Sum/2

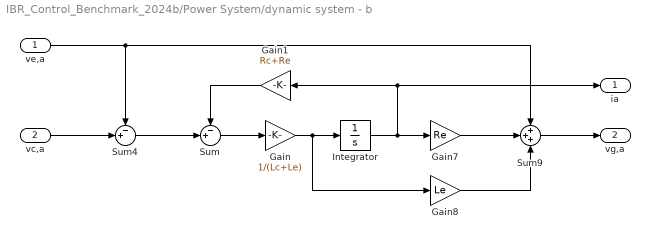
== system IBR_Control_Benchmark_2024b/Power System/dynamic system - b ==
  ve,a : Inport
  vc,a : Inport  Port=2
  Gain : Gain  Gain=1/(Lc+Le)
  Gain1 : Gain  Gain=Rc+Re
  Gain7 : Gain  Gain=Re
  Gain8 : Gain  Gain=Le
  Integrator : Integrator  InitialCondition=ib0
  Sum : Sum  Inputs=-+|
  Sum4 : Sum  Inputs=-+|
  Sum9 : Sum  Inputs=+++
  ia : Outport
  vg,a : Outport  Port=2
  wires:
  Gain/1 -> Integrator/1, Gain8/1
  Gain7/1 -> Sum9/2
  vc,a/1 -> Sum4/2
  Gain8/1 -> Sum9/3
  Integrator/1 -> ia/1, Gain1/1, Gain7/1
  ve,a/1 -> Sum9/1, Sum4/1
  Sum9/1 -> vg,a/1
  Sum/1 -> Gain/1
  Gain1/1 -> Sum/1
  Sum4/1 -> Sum/2

== system IBR_Control_Benchmark_2024b/Power System/dynamic system - c ==
  ve,a : Inport
  vc,a : Inport  Port=2
  Gain : Gain  Gain=1/(Lc+Le)
  Gain1 : Gain  Gain=Rc+Re
  Gain7 : Gain  Gain=Re
  Gain8 : Gain  Gain=Le
  Integrator : Integrator  InitialCondition=ic0
  Sum : Sum  Inputs=-+|
  Sum4 : Sum  Inputs=-+|
  Sum9 : Sum  Inputs=+++
  ia : Outport
  vg,a : Outport  Port=2
  wires:
  Gain/1 -> Integrator/1, Gain8/1
  Gain7/1 -> Sum9/2
  vc,a/1 -> Sum4/2
  Gain8/1 -> Sum9/3
  Integrator/1 -> ia/1, Gain1/1, Gain7/1
  ve,a/1 -> Sum9/1, Sum4/1
  Sum9/1 -> vg,a/1
  Sum/1 -> Gain/1
  Gain1/1 -> Sum/1
  Sum4/1 -> Sum/2

== system IBR_Control_Benchmark_2024b/IBR Control System/inverse park transformation/inverse park transformation matrix ==
  in:theta : Inport
  COS : Trigonometry  Operator=cos
  COS1 : Trigonometry  Operator=cos
  Gain : Gain  Gain=-1
  SIN : Trigonometry
  SIN1 : Trigonometry
  Vector Concatenate1 : Concatenate  Mode=Multidimensional array  ConcatenateDimension=2
  Vector Concatenate2 : Concatenate  Mode=Multidimensional array  ConcatenateDimension=2
  Vector Concatenate3 : Concatenate  Mode=Multidimensional array
  out:Tpark : Outport
  wires:
  Vector Concatenate2/1 -> Vector Concatenate3/2
  COS/1 -> Vector Concatenate1/1
  in:theta/1 -> COS1/1, SIN1/1, COS/1, SIN/1
  SIN/1 -> Gain/1
  Vector Concatenate1/1 -> Vector Concatenate3/1
  SIN1/1 -> Vector Concatenate2/1
  Vector Concatenate3/1 -> out:Tpark/1
  COS1/1 -> Vector Concatenate2/2
  Gain/1 -> Vector Concatenate1/2

== system IBR_Control_Benchmark_2024b/IBR Control System/park transformation/park transformation matrix ==
  in:theta : Inport
  COS : Trigonometry  Operator=cos
  COS1 : Trigonometry  Operator=cos
  Gain : Gain  Gain=-1
  SIN : Trigonometry
  SIN1 : Trigonometry
  Vector Concatenate1 : Concatenate  Mode=Multidimensional array  ConcatenateDimension=2
  Vector Concatenate2 : Concatenate  Mode=Multidimensional array  ConcatenateDimension=2
  Vector Concatenate3 : Concatenate  Mode=Multidimensional array
  out:Tpark : Outport
  wires:
  Vector Concatenate2/1 -> Vector Concatenate3/2
  COS/1 -> Vector Concatenate1/1
  in:theta/1 -> COS1/1, SIN1/1, COS/1, SIN/1
  SIN/1 -> Vector Concatenate1/2
  Vector Concatenate1/1 -> Vector Concatenate3/1
  Gain/1 -> Vector Concatenate2/1
  Vector Concatenate3/1 -> out:Tpark/1
  SIN1/1 -> Gain/1
  COS1/1 -> Vector Concatenate2/2
